simulink model "pidexample"  (R2014b)
settings: Solver=ode45  StartTime=0.0  StopTime=50.0  RelTol=1e-3
values from neighbouring files (symbols this model uses):
  m1 = ((I2*I3*I4)/(Rt2*Rt3*Cs))+(((Rt3*I4+Rt2*I1*I3*(I2+I4))/(Rt1*Rt2*Rt3*Cs)))    (= 24020)    [vars.m]
  m2 = (((I1+I3)*(I2*Rt2+I4*(Rt2+Rt3)))/(Rt2*Rt3*Cs))+((I1*I3*(Rt2+Rt3))/(Rt1*Rt3*Cs))    (= 3200)    [vars.m]
  m3 = (((I1+I3)*(Rt2+Rt3))/(Rt3*Cs))+((I1*I2*I4)/(Rt1*Rt2*Rt3))+((I1*I2*I3)/(Rt1*Rt2*Rt3))-((I1*I3*Rt2)/(Rt1*Rt3*Cs))    (= 15680)    [vars.m]
  s2 = ((Rt2*I1+Rt3*I1+Rt1*I2+Rt1*I3)/Cs1)+((I1*Rt3+I2*Rt3+Rt2*I3+Rt1*Rt2*Rt3+Rt1*I3)/Cs2)    (= 153)    [ssssss.m]
undefined symbols (not defined in the file or in its folder): s1
settings Model: Creator=Jacek  LastModifiedBy=Jacek

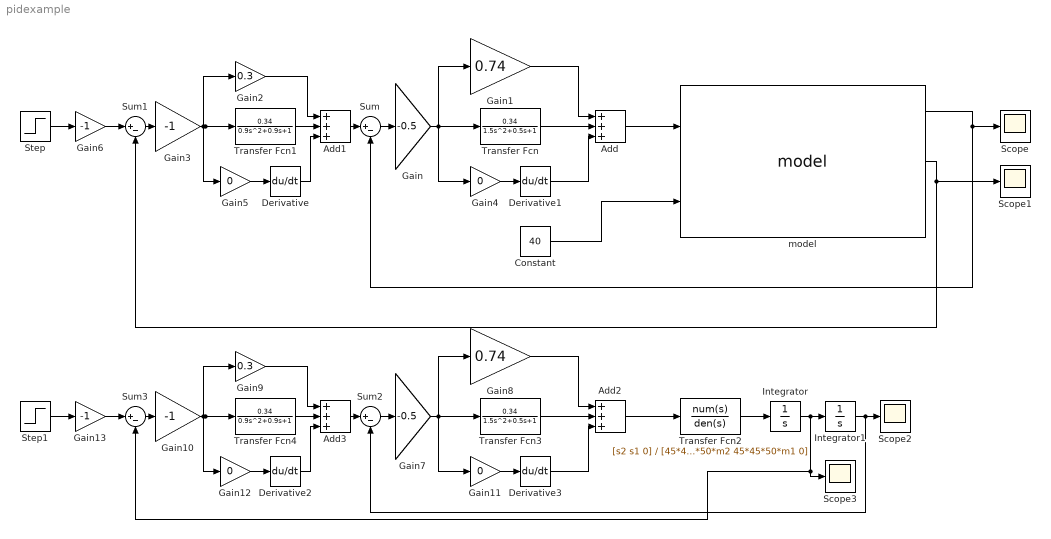
== system pidexample ==
  Add{,1..3} (4 alike) : Sum  Inputs=+++
  Constant : Constant  Value=40
  Derivative{,1..3} (4 alike) : Derivative
  Gain : Gain  Gain=-0.5
  Gain1 : Gain  Gain=0.74
  Gain{3,6,10,13} (4 alike) : Gain  Gain=-1
  Gain{4..5,11..12} (4 alike) : Gain  Gain=0
  Gain2 : Gain  Gain=0.3
  Gain7 : Gain  Gain=-0.5
  Gain8 : Gain  Gain=0.74
  Gain9 : Gain  Gain=0.3
  Integrator : Integrator
  Integrator1 : Integrator
  Scope{,1..3} (4 alike) : Scope
      Scope settings: YMin=9  YMax=11
      Scope2 settings: SaveName=ScopeData2
      Scope3 settings: SaveName=ScopeData3
  Step : Step  Time=0  After=1000  SampleTime=0
  Step1 : Step  Time=0  After=1000  SampleTime=0
  Sum{,1..3} (4 alike) : Sum  Inputs=|+-
  Transfer Fcn : TransferFcn  Numerator=[0.34]  Denominator=[1.5 0.5 1]
  Transfer Fcn1 : TransferFcn  Numerator=[0.34]  Denominator=[0.9 0.9 1]
  Transfer Fcn2 : TransferFcn  Numerator=[s2 s1 0]  Denominator=[45*45*50*m3 45*45*50*m2 45*45*50*m1 0]
  Transfer Fcn3 : TransferFcn  Numerator=[0.34]  Denominator=[1.5 0.5 1]
  Transfer Fcn4 : TransferFcn  Numerator=[0.34]  Denominator=[0.9 0.9 1]
  model : S-Function  FunctionName=model  EnableBusSupport=off
      mask Display: port_label('input',1,'Ein.'); port_label('input',2,'Fin.'); port_label('output',1,'Pout.'); port_label('output',2,'Vout.'); port_label('output',3,'DEBUG')
  wires:
  Add/1 -> model/1
  Transfer Fcn1/1 -> Add1/2
  Add1/1 -> Sum/1
  Gain4/1 -> Derivative1/1
  Gain/1 -> Transfer Fcn/1, Gain4/1, Gain1/1
  Derivative1/1 -> Add/3
  Transfer Fcn/1 -> Add/2
  Gain1/1 -> Add/1
  Sum/1 -> Gain/1
  Gain2/1 -> Add1/1
  Gain3/1 -> Transfer Fcn1/1, Gain5/1, Gain2/1
  Derivative/1 -> Add1/3
  Gain5/1 -> Derivative/1
  model/1 -> Scope/1, Sum/2
  model/2 -> Scope1/1, Sum1/2
  Constant/1 -> model/2
  Sum1/1 -> Gain3/1
  Gain6/1 -> Sum1/1
  Step/1 -> Gain6/1
  Transfer Fcn2/1 -> Integrator/1
  Add2/1 -> Transfer Fcn2/1
  Transfer Fcn4/1 -> Add3/2
  Add3/1 -> Sum2/1
  Gain11/1 -> Derivative3/1
  Gain7/1 -> Transfer Fcn3/1, Gain11/1, Gain8/1
  Derivative3/1 -> Add2/3
  Transfer Fcn3/1 -> Add2/2
  Gain8/1 -> Add2/1
  Sum2/1 -> Gain7/1
  Gain9/1 -> Add3/1
  Gain10/1 -> Transfer Fcn4/1, Gain12/1, Gain9/1
  Derivative2/1 -> Add3/3
  Gain12/1 -> Derivative2/1
  Integrator1/1 -> Sum2/2, Scope2/1
  Integrator/1 -> Sum3/2, Scope3/1, Integrator1/1
  Sum3/1 -> Gain10/1
  Gain13/1 -> Sum3/1
  Step1/1 -> Gain13/1
